simulink model "robot"  (R2022b)
settings: Solver=VariableStepAuto  StartTime=0.0  StopTime=20  RelTol=1e-3
undefined symbols (not defined in the file): m, r
settings Model: Creator=rplatz  LastModifiedBy=rplatz
settings ModelReferenceCC: EnableRefExpFcnMdlSchedulingChecks=on

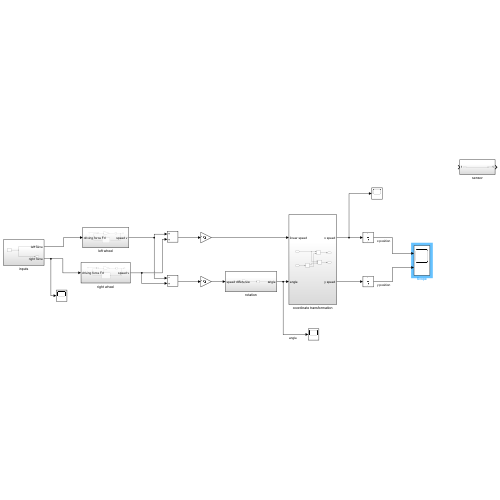
[thumbnail: Simulink's stored preview of the top-level diagram]
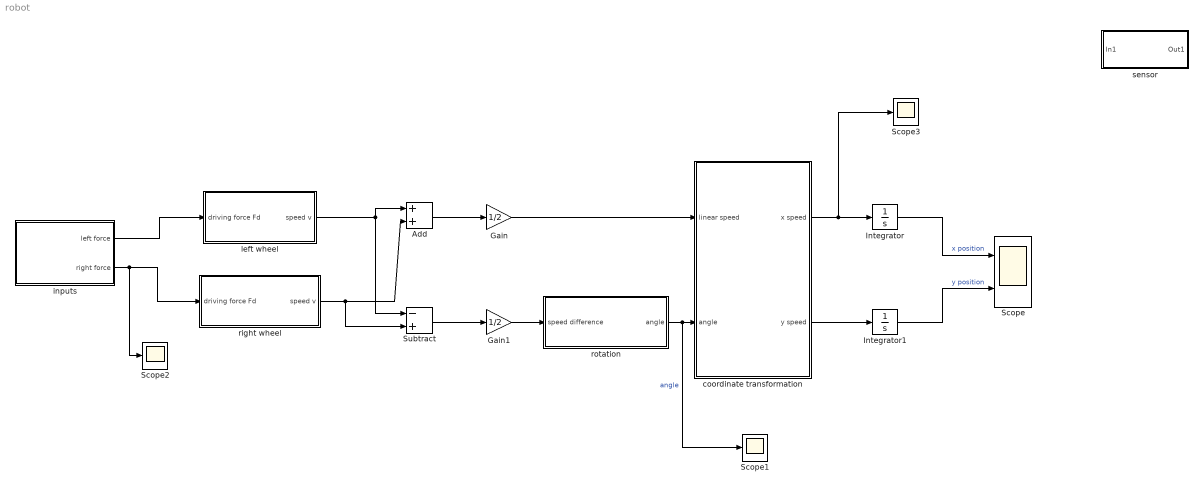
== system robot ==
  Add : Sum
  Gain : Gain  Gain=1/2
  Gain1 : Gain  Gain=1/2
  Integrator : Integrator
  Integrator1 : Integrator
  Scope : Scope  NumInputPorts=2
  Scope1 : Scope
  Scope2 : Scope
  Scope3 : Scope
  Subtract : Sum  Inputs=-+
  coordinate transformation : Subsystem
  inputs : Subsystem
  left wheel : Subsystem
  right wheel : Subsystem
  rotation : Subsystem
  sensor : Subsystem
  wires:
  coordinate transformation/1(x speed) -> Scope3/1, Integrator/1
  coordinate transformation/2(y speed) -> Integrator1/1
  inputs/1(left force) -> left wheel/1(driving force Fd)
  left wheel/1(speed v) -> Add/1, Subtract/1
  Add/1 -> Gain/1
  Subtract/1 -> Gain1/1
  Gain1/1 -> rotation/1(speed difference)
  rotation/1(angle) -> Scope1/1, coordinate transformation/2(angle)  "angle"
  Gain/1 -> coordinate transformation/1(linear speed)
  inputs/2(right force) -> Scope2/1, right wheel/1(driving force Fd)
  right wheel/1(speed v) -> Subtract/2, Add/2
  Integrator/1 -> Scope/1  "x position"
  Integrator1/1 -> Scope/2  "y position"

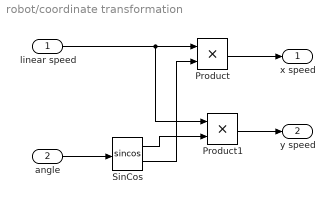
== system robot/coordinate transformation ==
  linear speed : Inport
  angle : Inport  Port=2
  Product : Product
  Product1 : Product
  SinCos : Trigonometry  Operator=sincos
  x speed : Outport
  y speed : Outport  Port=2
  wires:
  angle/1 -> SinCos/1
  linear speed/1 -> Product1/1, Product/1
  SinCos/2 -> Product/2
  SinCos/1 -> Product1/2
  Product1/1 -> y speed/1
  Product/1 -> x speed/1

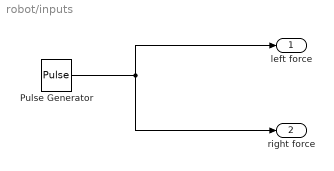
== system robot/inputs ==
  Pulse Generator : DiscretePulseGenerator  PulseType=Time based  Period=20  PulseWidth=15
  left force : Outport
  right force : Outport  Port=2
  wires:
  Pulse Generator/1 -> left force/1, right force/1

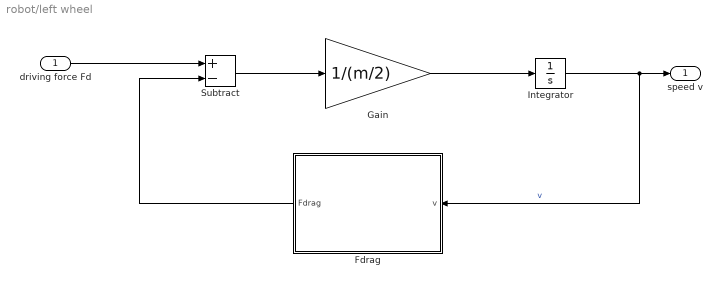
== system robot/left wheel ==
  driving force Fd : Inport
  Fdrag : MATLAB Function  TreatAsAtomicUnit=on
  Gain : Gain  Gain=1/(m/2)
  Integrator : Integrator
  Subtract : Sum  Inputs=+-
  speed v : Outport
  wires:
  driving force Fd/1 -> Subtract/1
  Fdrag/1(Fdrag) -> Subtract/2
  Subtract/1 -> Gain/1
  Gain/1 -> Integrator/1
  Integrator/1 -> Fdrag/1(v), speed v/1  "v"

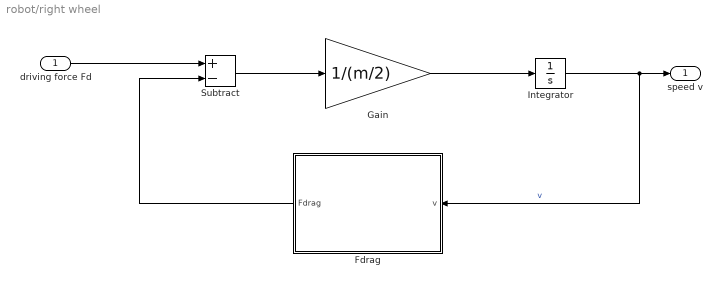
== system robot/right wheel ==
  driving force Fd : Inport
  Fdrag : MATLAB Function  TreatAsAtomicUnit=on
  Gain : Gain  Gain=1/(m/2)
  Integrator : Integrator
  Subtract : Sum  Inputs=+-
  speed v : Outport
  wires:
  Subtract/1 -> Gain/1
  Gain/1 -> Integrator/1
  driving force Fd/1 -> Subtract/1
  Integrator/1 -> Fdrag/1(v), speed v/1  "v"
  Fdrag/1(Fdrag) -> Subtract/2

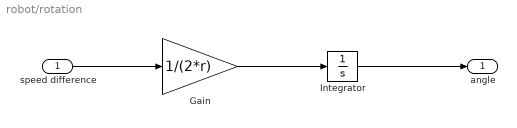
== system robot/rotation ==
  speed difference : Inport
  Gain : Gain  Gain=1/(2*r)
  Integrator : Integrator
  angle : Outport
  wires:
  Gain/1 -> Integrator/1
  Integrator/1 -> angle/1
  speed difference/1 -> Gain/1

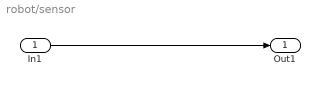
== system robot/sensor ==
  In1 : Inport
  Out1 : Outport
  wires:
  In1/1 -> Out1/1

== matlab function robot/left wheel/Fdrag ==
  data: v input; Fdrag output; k_drag parameter
function Fdrag = get_Fdrag(v,k_drag)

Fdrag = k_drag*v*abs(v);

== matlab function robot/right wheel/Fdrag ==
  data: v input; Fdrag output; k_drag parameter
function Fdrag = get_Fdrag(v,k_drag)

Fdrag = k_drag*v*abs(v);
